simulink model "Elevator"  (R2024b)
settings: Solver=VariableStepAuto  StartTime=0.0  StopTime=inf  RelTol=1e-3
settings Model: Creator=sunil  LastModifiedBy=sunil

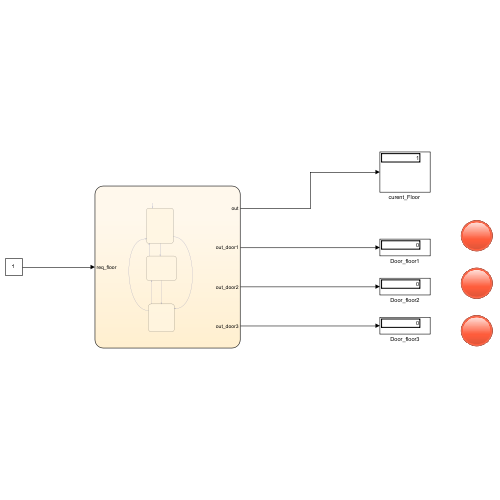
[thumbnail: Simulink's stored preview of the top-level diagram]
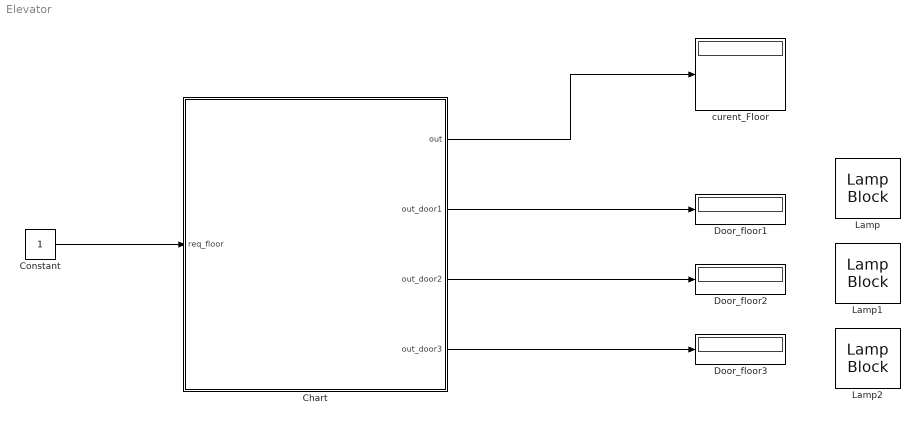
== system Elevator ==
  Chart : Stateflow chart  TreatAsAtomicUnit=on
  Constant : Constant
  Door_floor1 : Display
  Door_floor2 : Display
  Door_floor3 : Display
  Lamp : LampBlock  LabelPosition=Hide
  Lamp1 : LampBlock  LabelPosition=Hide
  Lamp2 : LampBlock  LabelPosition=Hide
  "curent_Floor " : Display
  wires:
  Constant/1 -> Chart/1(req_floor)
  Chart/2(out_door1) -> Door_floor1/1
  Chart/3(out_door2) -> Door_floor2/1
  Chart/4(out_door3) -> Door_floor3/1
  Chart/1(out) -> "curent_Floor "/1

== stateflow chart Elevator/Chart ==
  state Floor1
    entry:
    current_floor = 1;
    out= current_floor
    if (current_floor ==1)
    door_floor1 = 1;
    out_door1 = door_floor1;
    end
    during:
    if after(5, sec)
    door_floor1 = 0;
    out_door1 = door_floor1;
    end
    exit:
    door_floor1 = 0;
    out_door1 = door_floor1;
  state Floor2
    entry:
    current_floor = 2;
    out = current_floor
    door_floor1 = 0;
    door_floor2 = 1;
    out_door2 = door_floor2;
    during:
    if after(5, sec)
    door_floor2 = 0;
    out_door2 = door_floor2;
    end
  state Floor3_
    entry:
    current_floor = 3;
    out = current_floor
    door_floor3 = 1;
    out_door3 = door_floor3;
    during:
    if after(5, sec)
    door_floor3 = 0;
    out_door3 = door_floor3;
    end
  (default) -> Floor1
  Floor1 -> Floor3_ [order 2] : [req_floor==3]
  Floor3_ -> Floor1 [order 2] : [req_floor==1]
  Floor2 -> Floor1 [order 2] : [req_floor==1]
  Floor1 -> Floor2 [order 1] : [req_floor==2]
  Floor3_ -> Floor2 [order 1] : [req_floor==2]
  Floor2 -> Floor3_ [order 1] : [req_floor==3]
  data: out output; req_floor input; current_floor local; out_door1 output; out_door2 output; door_floor2 local; door_floor3 local; door_floor1 local; out_door3 output
